simulink model "PID_sldemo_absbrake"  (R2026a)
settings: Solver=FixedStepAuto  StopTime=25  FixedStep=0.01  MaxStep=.01  AbsTol=1e-6
PreLoadFcn:
  | % Load initialization data
  | 
  | sldemo_absdata;
StopFcn:
  |  if exist ('sldemo_absbrake_output')
  |  sldemo_absbrakeplots;
  |  end
values from neighbouring files (symbols this model uses):
  ctrl = 0    [ModelingAnAntiLockBrakingSystemExample.m]
undefined symbols (not defined in the file or in its folder): DiscIntNeverNeededParam, g, m, mu, Rr, v0
libraries: slpidlib x1
CloseFcn:
  | % Close the plots that are still open
  | h = findobj(0, 'Name', 'ABS Speeds');
  | if ~isempty(h),
  |   close(h);
  | end;
  | 
  | h = findobj(0, 'Name', 'ABS Slip');
  | if ~isempty(h),
  |   close(h);
  | end;
  | 
  | % Clear initial conditions data to avoid cluttering the workspace
  | 
  | clear g v0 Rr Kf m PBmax TB I slip mu ctrl h;
Description:
  | Modeling an Anti-Lock Braking System (ABS)
  | 
  | *Summary*
  | 
  | This example describes a simple model for an Anti-Lock Braking System
  | (ABS). The model simulates the dynamic behavior of a vehicle
  | under hard braking conditions. The model represents a single wheel, which
  | may be replicated a number of times to create a model for a multi-wheel
  | vehicle.
  | 
  | This model uses the signal logging feature in Simulink(R). You log signals to the
  | MATLAB(R) workspace where you can analyze and view them. You can view
  | the code in sldemo_absbrakeplots.m to see how this is done.
  | 
  | In this model, the wheel speed is calculated in a separate component
  | named sldemo_wheelspeed_absbrake.
  | This component is then referenced using a Model block.  Note that both the
  | top model and the referenced model use a variable step solver, so Simulink
  | will track zero-crossings in the referenced model.
settings Model: FPTRunName=Active  ModifiedByFormat=The MathWorks, Inc.  ExtModeTrigMode=oneshot  ExtModeArmWhenConnect=off  ExtModeAutoUpdateStatusClock=off  Creator=The MathWorks, Inc.  LastModifiedBy=The MathWorks, Inc.
settings DataIOCC: TimeSaveName=time  SignalLoggingName=sldemo_absbrake_output
settings OptimizationCC: UseDivisionForNetSlopeComputation=on  InlineInvariantSignals=on  StateBitsets=on  DataBitsets=on  EfficientFloat2IntCast=on  BufferReusableBoundary=off
settings DebuggingCC: SignalInfNanChecking=warning  SaveWithParameterizedLinksMsg=none  SigSpecEnsureSampleTimeMsg=none  IntegerOverflowMsg=error  UniqueDataStoreMsg=error  BusObjectLabelMismatch=none  AssertControl=DisableAll  SubsystemReferenceDiagnosticForUnitTest=warning  SFUndirectedBroadcastEventsDiag=error  IntegerSaturationMsg=none
settings HardwareCC: ProdHWDeviceType=32-bit Generic  TargetBitPerLong=64.0  TargetBitPerPointer=64.0  TargetBitPerSizeT=64.0  TargetBitPerPtrDiffT=64.0  TargetLongLongMode=on  TargetIntDivRoundTo=Zero  TargetEndianess=LittleEndian  TargetWordSize=64.0  TargetHWDeviceType=MATLAB Host
settings SFSimCC: CompileTimeRecursionLimit=0.0  EnableRuntimeRecursion=off
settings RTWCC: SystemTargetFile=ert.tlc  Description=Embedded Coder
settings CodeAppCC: IgnoreTestpoints=on  MATLABFcnDesc=on
settings ERTTargetCC: EnableSignedLeftShifts=off  EnableSignedRightShifts=off  DynamicArrayContainerType=coder::array  UtilityFuncGeneration=Shared location  GenerateSampleERTMain=on  SupportAbsoluteTime=off  ParenthesesLevel=Standards  CastingMode=Standards  GenerateSharedConstants=off
settings SimscapeCC: SimscapeNominalValues="[{\"value\":\"1\",\"unit\":\"A\"},{\"value\":\"1\",\"unit\":\"bar\"},{\"value\":\"1\",\"unit\":\"cm^2\"},{\"value\":\"1\",\"unit\":\"cm^3/s\"},{\"value\":\"1\",\"unit\":\"kJ/kg\"},{\"value\":\"1\",\"unit\":\"kW\"},{\"value\":\"1\",\"unit\":\"l\"},{\"value\":\"1\",\"unit\":\"N\"},{\"value\":\"1\",\"unit\":\"N*m\"},{\"value\":\"1\",\"unit\":\"V\"}]"  SimscapeLogType=none  SimscapeLogDataHistory=5000.0

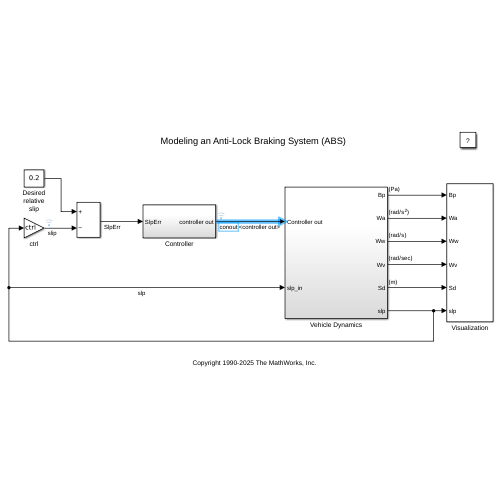
[thumbnail: Simulink's stored preview of the top-level diagram]
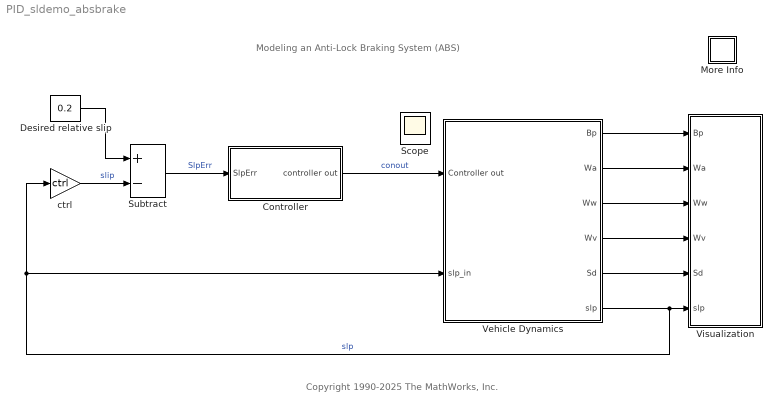
== system PID_sldemo_absbrake ==
  note: Modeling an Anti-Lock Braking System (ABS)
  note: Copyright 1990-2025 The MathWorks, Inc.
  Controller : Subsystem
  Desired relative slip : Constant  Value=0.2
  More Info : Subsystem
      settings: OpenFcn=showExample('simulink_automotive/ModelingAnAntiLockBrakingSystemExample')
      mask Display: disp('?')
  Subtract : Sum  Inputs=+-
  Vehicle Dynamics : Subsystem
  Visualization : Subsystem
  ctrl : Gain  Gain=ctrl
  Scope : Scope
      settings: ActiveDisplayYMinimum=-8.8  ActiveDisplayYMaximum=79.2
  wires:
  Subtract/1 -> Controller/1(SlpErr)  "SlpErr"
  Desired relative slip/1 -> Subtract/1
  ctrl/1 -> Subtract/2  "slip"
  Vehicle Dynamics/6(slp) -> ctrl/1, Vehicle Dynamics/2(slp_in), Visualization/6(slp)  "slp"
  Controller/1(controller out) -> Vehicle Dynamics/1(Controller out)  "conout"
  Vehicle Dynamics/1(Bp) -> Visualization/1(Bp)
  Vehicle Dynamics/2(Wa) -> Visualization/2(Wa)
  Vehicle Dynamics/3(Ww) -> Visualization/3(Ww)
  Vehicle Dynamics/4(Wv) -> Visualization/4(Wv)
  Vehicle Dynamics/5(Sd) -> Visualization/5(Sd)

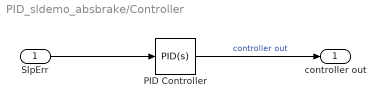
== system PID_sldemo_absbrake/Controller ==
  SlpErr : Inport
  PID Controller : slpidlib/PID Controller  Controller=PID  Form=Parallel  TimeDomain=Continuous-time  UseExternalTs=off  SampleTime=-1  IntegratorMethod=Forward Euler  FilterMethod=Forward Euler  ControllerParametersSource=internal  P=25  I=0.05  UseKiTs=off  D=0.3  UseExternalDerivativeSource=off  N=100  UseFilter=on  TunerSelectOption=Transfer Function Based (PID Tuner App)  InitialConditionSource=internal  InitialConditionForIntegrator=0  InitialConditionForFilter=0  DifferentiatorICPrevScaledInput=0  ExternalReset=none  TrackingMode=off  Kt=1  LimitOutput=on  SatLimitsSource=internal  UpperSaturationLimit=inf  LowerSaturationLimit=-inf  LinearizeAsGain=on  AntiWindupMode=clamping  Kb=1  LimitIntegrator=on  UpperIntegratorSaturationLimit=inf  LowerIntegratorSaturationLimit=-inf  POutMin=[]  POutMax=[]  IOutMin=[]  IOutMax=[]  DOutMin=[]  DOutMax=[]  NOutMin=[]  NOutMax=[]  SumOutMin=[]  SumOutMax=[]  SaturationOutMin=[]  SaturationOutMax=[]  PParamMin=[]  PParamMax=[]  IParamMin=[]  IParamMax=[]  DParamMin=[]  DParamMax=[]  NParamMin=[]  NParamMax=[]  KbParamMin=[]  KbParamMax=[]  KtParamMin=[]  KtParamMax=[]  KbOutMin=[]  KbOutMax=[]  KtOutMin=[]  KtOutMax=[]  IntegratorOutMin=[]  IntegratorOutMax=[]  FilterOutMin=[]  FilterOutMax=[]  SumI1OutMin=[]  SumI1OutMax=[]  SumI2OutMin=[]  SumI2OutMax=[]  SumI3OutMin=[]  SumI3OutMax=[]  SumI4OutMin=[]  SumI4OutMax=[]  SumDOutMin=[]  SumDOutMax=[]  DifferentiatorOutMin=[]  DifferentiatorOutMax=[]  FilterDiffOutCoefMin=[]  FilterDiffOutCoefMax=[]  ReciprocalOutMin=[]  ReciprocalOutMax=[]  SumDenOutMin=[]  SumDenOutMax=[]  SumNumOutMin=[]  SumNumOutMax=[]  DivideOutMin=[]  DivideOutMax=[]  UdiffTsProdOutMin=[]  UdiffTsProdOutMax=[]  NTsProdOutMin=[]  NTsProdOutMax=[]  UintegralTsProdOutMin=[]  UintegralTsProdOutMax=[]  UngainTsProdOutMin=[]  UngainTsProdOutMax=[]  ClampingZeroOutDataTypeStr=Inherit: Inherit via back propagation  ClampingZeroOutMin=[]  ClampingZeroOutMax=[]  FilterDenConstantOutDataTypeStr=Inherit: Inherit via back propagation  FilterDenConstantOutMin=[]  FilterDenConstantOutMax=[]  PCopyOutDataTypeStr=Inherit: Inherit via back propagation  PCopyOutMin=[]  PCopyOutMax=[]  NCopyOutDataTypeStr=Inherit: Inherit via back propagation  NCopyOutMin=[]  NCopyOutMax=[]  IntegratorContinuousStateAttributes=''  IntegratorStateMustResolveToSignalObject=off  IntegratorRTWStateStorageClass=Auto  FilterContinuousStateAttributes=''  FilterStateMustResolveToSignalObject=off  FilterRTWStateStorageClass=Auto  ParallelPVariant=InternalParameters  IdealPVariant=Disabled  IVariant=InternalParameters  DVariant=InternalParameters  IntegratorVariant=Continuous  SatVariant=Enabled  AWVariant=ContClampingParallel  PCopyVariant=Disabled  TRVariant=Disabled  FdbkBlocksVariant=Forward  IdealPFdbkVariant=Disabled  SatFdbkVariant=Disabled  DerivativeFilterVariant=ContFilter  NVariant=InternalParameters  NCopyVariant=Disabled  FilterICVariant=InternalICsFilter  IntegratorICVariant=InternalICs  ExternalResetVariant=Disabled  TRSumVariant=Passthrough  SumFdbkVariant=Disabled  SumVariant=Sum_PID  TsampFilterVariant=InternalTs  TsampNgainVariant=Passthrough  TsampIntegralVariant=Disabled_SignalSpec  ExternalSaturationOutDataTypeStr=Inherit: Same as second input  DerivativeSourceVariant=ErrorSignal  PreIntVariant=InternalPreInt
  controller out : Outport
  wires:
  PID Controller/1 -> controller out/1  "controller out"
  SlpErr/1 -> PID Controller/1

== system PID_sldemo_absbrake/More Info ==

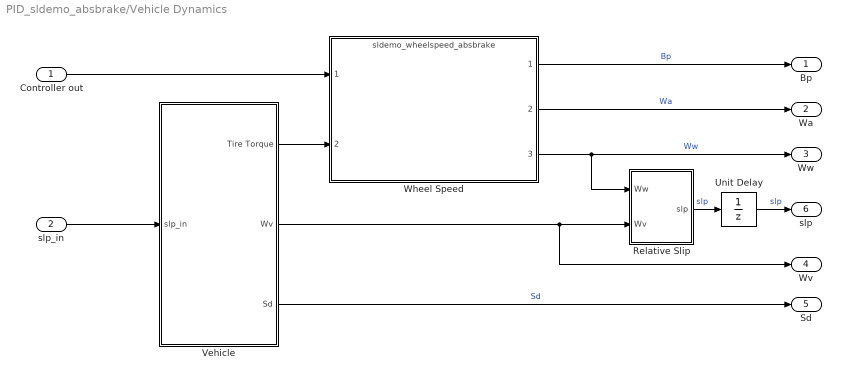
== system PID_sldemo_absbrake/Vehicle Dynamics ==
  Controller out : Inport
  slp_in : Inport  Port=2
  Relative Slip : Subsystem
  Unit Delay : UnitDelay  SampleTime=-1
  "Vehicle  " : Subsystem
  Wheel Speed : ModelReference  ModelNameDialog=sldemo_wheelspeed_absbrake.slx  SimulationMode=Normal  ModelReferenceVersion=12.4
  Bp : Outport
  Wa : Outport  Port=2
  Ww : Outport  Port=3
  Wv : Outport  Port=4
  Sd : Outport  Port=5
  slp : Outport  Port=6
  wires:
  Wheel Speed/3 -> Relative Slip/1(Ww), Ww/1  "Ww"
  "Vehicle  "/2(Wv) -> Wv/1, Relative Slip/2(Wv)
  "Vehicle  "/1(Tire Torque) -> Wheel Speed/2
  "Vehicle  "/3(Sd) -> Sd/1  "Sd"
  Relative Slip/1(slp) -> Unit Delay/1  "slp"
  Controller out/1 -> Wheel Speed/1
  Wheel Speed/1 -> Bp/1  "Bp"
  slp_in/1 -> "Vehicle  "/1(slp_in)
  Wheel Speed/2 -> Wa/1  "Wa"
  Unit Delay/1 -> slp/1  "slp"

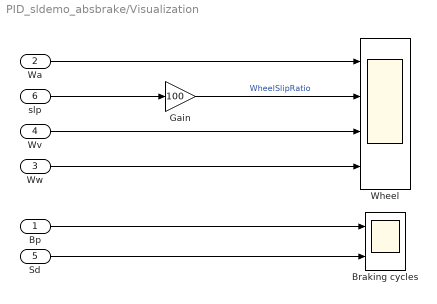
== system PID_sldemo_absbrake/Visualization ==
  Bp : Inport
  Wa : Inport  Port=2
  Ww : Inport  Port=3
  Wv : Inport  Port=4
  Sd : Inport  Port=5
  slp : Inport  Port=6
  Braking cycles : Scope  NumInputPorts=2
      settings: ActiveDisplayYMinimum=-90.25511  ActiveDisplayYMaximum=812.29596
  Gain : Gain  Gain=100
  Wheel : Scope  NumInputPorts=4
      settings: ActiveDisplayYMinimum=-27.40083  ActiveDisplayYMaximum=12.545
  wires:
  Bp/1 -> Braking cycles/1
  Wa/1 -> Wheel/1
  Ww/1 -> Wheel/4
  Sd/1 -> Braking cycles/2
  Wv/1 -> Wheel/3
  Gain/1 -> Wheel/2  "WheelSlipRatio"
  slp/1 -> Gain/1

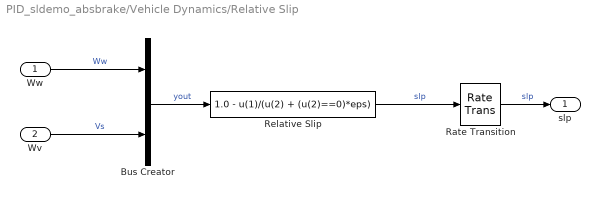
== system PID_sldemo_absbrake/Vehicle Dynamics/Relative Slip ==
  Ww : Inport
  Wv : Inport  Port=2
  Bus Creator : BusCreator  Inputs=2
  Rate Transition : RateTransition  OutPortSampleTimeOpt=Inherit
  Relative Slip : Fcn  Expr=1.0 - u(1)/(u(2) + (u(2)==0)*eps)
  slp : Outport
  wires:
  Bus Creator/1 -> Relative Slip/1  "yout"
  Relative Slip/1 -> Rate Transition/1  "slp"
  Ww/1 -> Bus Creator/1  "Ww"
  Wv/1 -> Bus Creator/2  "Vs"
  Rate Transition/1 -> slp/1  "slp"

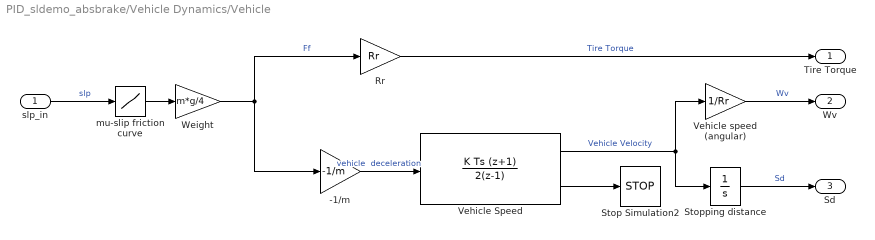
== system PID_sldemo_absbrake/Vehicle Dynamics/Vehicle   ==
  slp_in : Inport
  -1/m : Gain  Gain=-1/m  SaturateOnIntegerOverflow=on  OutDataTypeStr=Inherit: Same as input  ParamDataTypeStr=Inherit: Same as input
  Rr : Gain  Gain=Rr  SaturateOnIntegerOverflow=on  OutDataTypeStr=Inherit: Same as input  ParamDataTypeStr=Inherit: Same as input
  Stop Simulation2 : Stop
  Stopping distance : Integrator  UpperSaturationLimit=1000  LowerSaturationLimit=0
  Vehicle Speed : DiscreteIntegrator  IntegratorMethod=Integration: Trapezoidal  InitialCondition=v0  SampleTime=-1  LimitOutput=on  UpperSaturationLimit=1000  LowerSaturationLimit=0  ShowSaturationPort=on  ICPrevOutput=DiscIntNeverNeededParam  ICPrevScaledInput=DiscIntNeverNeededParam
  Vehicle speed (angular) : Gain  Gain=1/Rr  SaturateOnIntegerOverflow=on  OutDataTypeStr=Inherit: Same as input  ParamDataTypeStr=Inherit: Same as input
  Weight : Gain  Gain=m*g/4  SaturateOnIntegerOverflow=on  OutDataTypeStr=Inherit: Same as input  ParamDataTypeStr=Inherit: Same as input
  mu-slip friction curve : Lookup_n-D  NumberOfTableDimensions=1  BreakpointsForDimension1=[0 0.05 0.1 0.15000000000000002 0.2 0.25 0.30000000000000004 0.35000000000000003 0.4 0.45 0.5 0.55 0.6 0.64999999999999991 0.7 0.75 0.8 0.85 0.9 0.95 1]  Table=mu  SaturateOnIntegerOverflow=on
  Tire Torque : Outport  Unit=N*m
  Wv : Outport  Port=2  Unit=rad/sec
  Sd : Outport  Port=3  Unit=m
  wires:
  slp_in/1 -> mu-slip friction curve/1  "slp"
  Rr/1 -> Tire Torque/1  "Tire Torque"
  -1/m/1 -> Vehicle Speed/1  "vehicle  deceleration"
  Vehicle speed (angular)/1 -> Wv/1  "Wv"
  Stopping distance/1 -> Sd/1  "Sd"
  Weight/1 -> -1/m/1, Rr/1  "Ff"
  mu-slip friction curve/1 -> Weight/1
  Vehicle Speed/1 -> Stopping distance/1, Vehicle speed (angular)/1  "Vehicle Velocity"
  Vehicle Speed/2 -> Stop Simulation2/1
